simulink model "Simulink_Timer"  (R2018b)
settings: Solver=FixedStepDiscrete  StartTime=0.0  StopTime=10.0  FixedStep=0.001  RelTol=1e-3
libraries: simulink x2, GPIO_Lib x1, STM32_Config_Lib x1, TIMERS_Lib x1
settings Model: Creator=yangy  LastModifiedBy=yangy
settings OptimizationCC: DefaultParameterBehavior=Inlined  EnhancedBackFolding=on  PassReuseOutputArgsAs=Individual arguments  OptimizeBlockOrder=speed  DifferentSizesBufferReuse=on  OptimizationCustomize=off
settings DebuggingCC: ParameterTunabilityLossMsg=error
settings HardwareCC: ProdBitPerPointer=32  ProdBitPerSizeT=32  ProdBitPerPtrDiffT=32  ProdLargestAtomicInteger=Integer  ProdWordSize=32  ProdHWDeviceType=STM32CortexM
settings SFSimCC: MATLABDynamicMemAlloc=off
settings RTWCC: SystemTargetFile=stm32.tlc  TemplateMakefile=stm32.tmf  Description=stm32 (Embedded Target)  GenerateReport=on  IncludeHyperlinkInReport=on  GenerateTraceInfo=on  GenerateTraceReport=on  GenerateTraceReportSl=on  GenerateTraceReportSf=on  GenerateTraceReportEml=on
settings CodeAppCC: ForceParamTrailComments=on  IgnoreCustomStorageClasses=off  MaxIdLength=64  OperatorAnnotations=on  SimulinkDataObjDesc=on  SFDataObjDesc=on  CustomSymbolStrType=$N$R$M  SimulinkBlockComments=off
settings STFCustomTargetCC: TargetLangStandard=C99 (ISO)  CodeReplacementLibrary=ARM CMSIS SIN COS  MultiwordLength=256  ParMdlRefBuildCompliant=on  IncludeMdlTerminateFcn=off  CombineOutputUpdateFcns=on  ERTCustomFileBanners=on  SupportContinuousTime=off  SupportNonInlinedSFcns=off  RemoveResetFunc=on  MATLABClassNameForMDSCustomization=Simulink.SoftwareTarget.ERTCustomization  SystemTargetFile=stm32.tlc
settings ERTTargetCC: TargetLangStandard=C99 (ISO)  CodeReplacementLibrary=ARM CMSIS SIN COS  CompOptLevelCompliant=off  ConcurrentExecutionCompliant=off  IncludeMdlTerminateFcn=off  ModelStepFunctionPrototypeControlCompliant=off  CPPClassGenCompliant=off  UseToolchainInfoCompliant=off  ExtModeStaticAllocSize=256  ExtModeMexFile=ext_serial_win32_comm  ExtModeMexArgs=0,1,115200,10  InlinedParameterPlacement=NonHierarchical  ERTSrcFileBannerTemplate=sourceFileTemplate.cgt  ERTHdrFileBannerTemplate=sourceFileTemplate.cgt  ERTDataSrcFileTemplate=sourceFileTemplate.cgt  ERTDataHdrFileTemplate=sourceFileTemplate.cgt  ERTCustomFileTemplate=customRoutineProcess.tlc

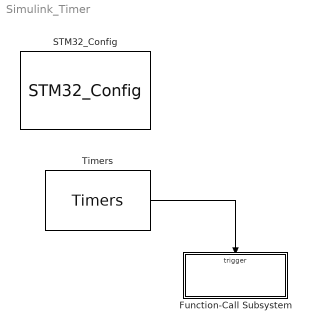
== system Simulink_Timer ==
  Function-Call Subsystem : Subsystem  TreatAsAtomicUnit=on
  STM32_Config : STM32_Config_Lib/STM32_Config  Priority=0  Project_Path=.\Simulink_Timer\  Config_File=Simulink_Timer.ioc  MCU_Name=STM32F405RGTx
      settings: SourceProductName=Target Support Package - STM32 Adapter
  Timers : TIMERS_Lib/Timers  currentTIM=TIM6  TIM_Name=TIM6  sysUsingTimer=off  TIM_APBClock=16000000  TIM_Set_Clk=off  TIM_Prescaler=83  TIM_Clock=190476.19  Variable_frequency=off  TIM_Set_OutFreq=off  TIM_ARR=1  Output_frequency=190476.19  Repetition_counter=0  TIM_Mode=Up  TIM_DMA=none  TIM_IRQ=off  TIM_IRQ_ONLY=on  TIM_UP=on  TIM_TRG=off  TIM_COM=off  TIM_BRK=off  NbTIM=1  CH1_enable=off  CH1N_enable=off  CH1_type=Unknown  CH1_DMA=off  CH1_int=off  CH1_edge=Rising  CH1_div=1  CH1_variable_duty=off  CH1_set_pulse=off  CH1_output_duty=0.00  CH1_pulse=0  CH2_enable=off  CH2N_enable=off  CH2_type=Unknown  CH2_DMA=off  CH2_int=off  CH2_edge=Rising  CH2_div=1  CH2_variable_duty=off  CH2_set_pulse=off  CH2_output_duty=0.00  CH2_pulse=0  CH3_enable=off  CH3N_enable=off  CH3_type=Unknown  CH3_DMA=off  CH3_int=off  CH3_edge=Rising  CH3_div=1  CH3_variable_duty=off  CH3_set_pulse=off  CH3_output_duty=0.00  CH3_pulse=0  CH4_enable=off  CH4N_enable=off  CH4_type=Unknown  CH4_DMA=off  CH4_int=off  CH4_edge=Rising  CH4_div=1  CH4_variable_duty=off  CH4_set_pulse=off  CH4_output_duty=0.00  CH4_pulse=0
      settings: SourceProductName=Target Support Package - STM32 Adapter
  wires:
  Timers/1 -> Function-Call Subsystem/Trigger

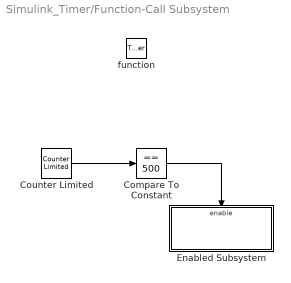
== system Simulink_Timer/Function-Call Subsystem ==
  function : TriggerPort  TriggerType=function-call  VariantControl=Variant
  Compare To Constant : simulink/Logic and Bit Operations/Compare To Constant  relop===  const=500  OutDataTypeStr=boolean
  Counter Limited : simulink/Sources/Counter Limited  uplimit=500  tsamp=-1
  Enabled Subsystem : Subsystem  TreatAsAtomicUnit=on
  wires:
  Counter Limited/1 -> Compare To Constant/1
  Compare To Constant/1 -> Enabled Subsystem/Enable

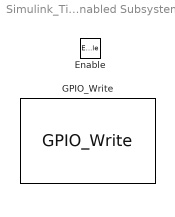
== system Simulink_Timer/Function-Call Subsystem/Enabled Subsystem ==
  Enable : EnablePort
  GPIO_Write : GPIO_Lib/GPIO_Write  Port_name=GPIOC  Pin0=on  Toggle_Pin0=on  Pin1=off  Toggle_Pin1=off  Pin2=off  Toggle_Pin2=off  Pin3=off  Toggle_Pin3=off  Pin4=off  Toggle_Pin4=off  Pin5=off  Toggle_Pin5=off  Pin6=off  Toggle_Pin6=off  Pin7=off  Toggle_Pin7=off  Pin8=off  Toggle_Pin8=off  Pin9=off  Toggle_Pin9=off  Pin10=off  Toggle_Pin10=off  Pin11=off  Toggle_Pin11=off  Pin12=off  Toggle_Pin12=off  Pin13=off  Toggle_Pin13=off  Pin14=off  Toggle_Pin14=off  Pin15=off  Toggle_Pin15=off  PinList="GPIOC0  1"
      settings: SourceProductName=Target Support Package - STM32 Adapter
